simulink model "Thesis_VehicleModel_MPC_ECMS"  (R2018b)
settings: Solver=FixedStepAuto  StartTime=0.0  StopTime=10  FixedStep=0.01  RelTol=1e-5
PostLoadFcn:
  | , if any(exist('dsrtsu_mdlpostloadfcn', 'file') == [2, 3, 6]), try dsrtsu_mdlpostloadfcn('Execute', bdroot); catch fprintf('Error in PostLoadFcn (dsrtsu_mdlpostloadfcn) for model "%s":\n %s\n', bdroot, lasterr); end, end,
InitFcn:
  | clc;clear all;
model workspace (MAT data in the model file):
  MDL.BatteryModel.AccyLoad = 600
  MDL.BatteryModel.Voc = 340
  MDL.BatteryModel.Rint = 0.08
  MDL.BatteryModel.Ecap = 8.8
  MDL.BatteryModel.SOCi = 0.5
  MDL.BrakeSys.MaxBrakeForce = 10000
  MDL.BrakeSys.RegenFraction = 0.55
  MDL.Driveline.TFRatio = 3.5
  MDL.Driveline.MaxTrac = 8000
  MDL.Driveline.BrakeGain = 500
  MDL.Driveline.Spinloss = 3.6
  MDL.EngineModel.C0 = 6760
  MDL.EngineModel.C1 = 1.32
  MDL.EngineModel.C2 = 4.2e-06
  MDL.EngineModel.LHV = 44400
  MDL.EngineModel.MaxOutPwr = 73000
  MDL.EngineModel.EngStartEnergy = 0
  MDL.EngineModel.AccyLoad = 600
  MDL.EngineModel.EffMapData = [800  800  800  800  800  800  800  800  800  800; 700  700  700  700  700  700  700  700  700  700; 600  600  600  600  600  600  600  600  600  600; 400  400  400  400  400  400  400  400  400  400; 275  275  275  275  275  275  278  280  285  290; 255  255  255  255  255  258  260  265  270  275; 245  244  243  243  244  245  248  250  260  265; 235  234  234  236  238  239  240  242  246  252; 225  222  221  223  226  228  230  232  242  247; 225  223  220  215  218  221  225  232  240  244; 227  226  221  216  218  220  226  232  242  244; 230  228  226  225  222  224  226  232  240  243; 235  234  228  226  226  227  229  234  241  244; 240  237  234  230  228  229  230  235  240  244; 245  242  240  235  232  231  235  240  242  244; 248  246  244  242  234  235  241  246  250  252]
  MDL.EngineModel.EffMapRPM = [800 1000 1500 2000 2500 3000 3500 4000 4500 5000]
  MDL.EngineModel.EffMapTorque = [0 10 20 30 40 50 60 70 80 90 100 110 120 130 135 150]
  MDL.GeneratorModel.C0 = 600
  MDL.GeneratorModel.C1 = 0.033
  MDL.GeneratorModel.C2 = 8e-07
  MDL.GeneratorModel.PeakMechPwr = 50000
  MDL.GeneratorModel.ContMechPwr = 25000
  MDL.HVSCModel.TargetSOC = 0.45
  MDL.HVSCModel.SOC_gain = 100000
  MDL.LHV = 46400
  MDL.MotorModel.EtoWRatio = 0.98
  MDL.MotorModel.MaxPwrOut = 80000
  MDL.MotorModel.MaxTorque = 240
  MDL.MotorModel.MaxWhlSpd = 600
  MDL.MotorModel.EffMapTorque = [0 50 75 100 125 150 175 200 240]
  MDL.MotorModel.EffMapRPM = [0 500 1000 1250 1500 1750 2000 2250 2500 2750 3000 3250 3500 3750 4000 4250 4500 5000]
  MDL.MotorModel.EffMapData = [0.8  0.815  0.82  0.825  0.83  0.83  0.84  0.84  0.84  0.84  0.84  0.84  0.84  0.83  0.82  0.81  0.8  0.76; 0.83  0.87  0.9  0.865  0.88  0.92  0.92  0.92  0.92  0.92  0.92  0.92  0.92  0.915  0.9  0.86  0.85  0.82; 0.83  0.88  0.94  0.945  0.948  0.95  0.96  0.96  0.96  0.956  0.95  0.95  0.948  0.946  0.945  0.938  0.9  0.85; 0.82  0.88  0.94  0.948  0.95  0.96  0.96  0.96  0.96  0.96  0.96  0.96  0.95  0.955  0.95  0.945  0.94  0.86; 0.81  0.88  0.94  0.95  0.958  0.96  0.96  0.96  0.96  0.96  0.96  0.96  0.958  0.954  0.952  0.952  0.948  0.9; 0.81  0.86  0.94  0.95  0.95  0.95  0.95  0.95  0.95  0.95  0.95  0.95  0.95  0.96  0.95  0.948  0.94  0.94; 0.8  0.886  0.91  0.94  0.945  0.948  0.946  0.944  0.944  0.948  0.947  0.946  0.9455  0.945  0.944  0.943  0.942  0.941; 0.79  0.84  0.9  0.92  0.93  0.94  0.94  0.94  0.94  0.94  0.94  0.94  0.94  0.94  0.94  0.94  0.94  0.94; 0.77  0.81  0.86  0.86  0.86  0.86  0.86  0.86  0.86  0.86  0.86  0.86  0.86  0.86  0.86  0.86  0.86  0.86]
  MDL.Tire.Miu = 0.9
  MDL.Tire.Caf = 39000
  MDL.Tire.Car = 39000
  MDL.Tire.ContactPatch = 0.0003
  MDL.Tire.EffectiveRadius = 0.31
  MDL.Tire.Inertia = 0.9182
  MDL.Tire.c_rr = 0.01
  MDL.Tire.RelaxationLength = 0.248
  MDL.VehicleDynamics.M = 1500
  MDL.VehicleDynamics.Mi = 1560
  MDL.VehicleDynamics.CdA = 0.76
  MDL.VehicleDynamics.rho = 1.2
  MDL.VehicleDynamics.grade = 0
  MDL.VehicleDynamics.g = 9.81
  MDL.VehicleDynamics.V_i = 0
  MDL.VehicleDynamics.FrontLength = 1.524
  MDL.VehicleDynamics.RearLength = 1.2192
  MDL.VehicleDynamics.WheelBase = 2.7432
  MDL.VehicleDynamics.Inertia = 3000
  MDL.VehicleDynamics.HeightofCD = 0.32
  MDL.VehicleDynamics.HeightofCG = 0.3
  MDL.ThrottleController.KFA = [0  1; -0.3425  -5.0685]
  MDL.ThrottleController.KFB = [0; 904.1096]
  MDL.ThrottleController.KFC = [1 0]
  MDL.ThrottleController.KFL = [3.2; -0.2946]
values from neighbouring files (symbols this model uses):
  MDL =     [MDL.mat]
libraries: simulink x14, rtican x9, autolibshared x1, mpclib x1
(part 1 of 5)
settings Model: DSRTSU_INTERNAL_RTI_VER=510  DSRTSU_INTERNAL_RTI_TYPE=rti1006  RTICANMMDATA=struct('GeneralSetupData',struct('modelroot','C:\Users\UWECOCAR3\Desktop\YD_Thesis_dSPACE_Model','generalsettings',struct('filesettings',struct('destfolder',struct('Name','RTICANMM_FILES','Check',1),'buildfolder',struct('Name','.','Check',1),'AbsDestfolder',struct('Name','C:\Users\UWECOCAR3\Desktop\YD_Thesis_dSPACE_Model\RTICANMM_FILES'),'AbsBuildfolder',struct('Name','C:\Users\UWECOCAR3\Desktop\YD_Thesis_dSPACE_Model'))),'options',struct('addpaths',1,'rmpaths',1,'addtrcexclusion',logical(1),'cannavigator',struct('checkmonitoring',0),'show_usrtrc',0,'use_usrtrc',0),'advanced',struct('options',[1 1 1 1 1 1 1 1 1 1 1 1 1 1 1 1 1 1 1 1 1 1 1 1 1 1 1 1 1 1 1 1 1 1 1 1 1 1 1 1 1 1 1 1 1 1 1 1 1 1 1 1 1 1 1 1 1 1 1 1 1 1 1 1 1 1 1 1 1 1 1 1 1 1 1 1 1 1 1 1 1 1 1 1 1 1 1 1 1 1 1 1 1 1 1 1 1 1 1 1]),'MPSetup',{{}},'modelname','Thesis_VehicleModel_Integrate_Powertrain_17b','block','Thesis_VehicleModel_Integrate_Powertrain_17b'))  DSRTSU_INTERNAL_RTIFLEXRAYCONFIG=110  DSRTSU_INTERNAL_RTIFPGA=110  Creator=lyd21  LastModifiedBy=lyd21
settings SolverCC: ZeroCrossAlgorithm=Adaptive
settings OptimizationCC: BlockReduction=off
settings DebuggingCC: MaxConsecutiveZCsMsg=none  IgnoredZcDiagnostic=none
settings HardwareCC: ProdBitPerPointer=32  ProdBitPerSizeT=32  ProdBitPerPtrDiffT=32  ProdLargestAtomicInteger=Integer  ProdWordSize=32  ProdHWDeviceType=Custom Processor->Custom  TargetIntDivRoundTo=Zero  TargetEndianess=LittleEndian  TargetHWDeviceType=Custom Processor->Custom
settings SFSimCC: SimUseLocalCustomCode=off  MATLABDynamicMemAlloc=off
settings RTWCC: Description=Generic Real-Time Target  RTWUseLocalCustomCode=off
settings GRTTargetCC: TargetLangStandard=C89/C90 (ANSI)

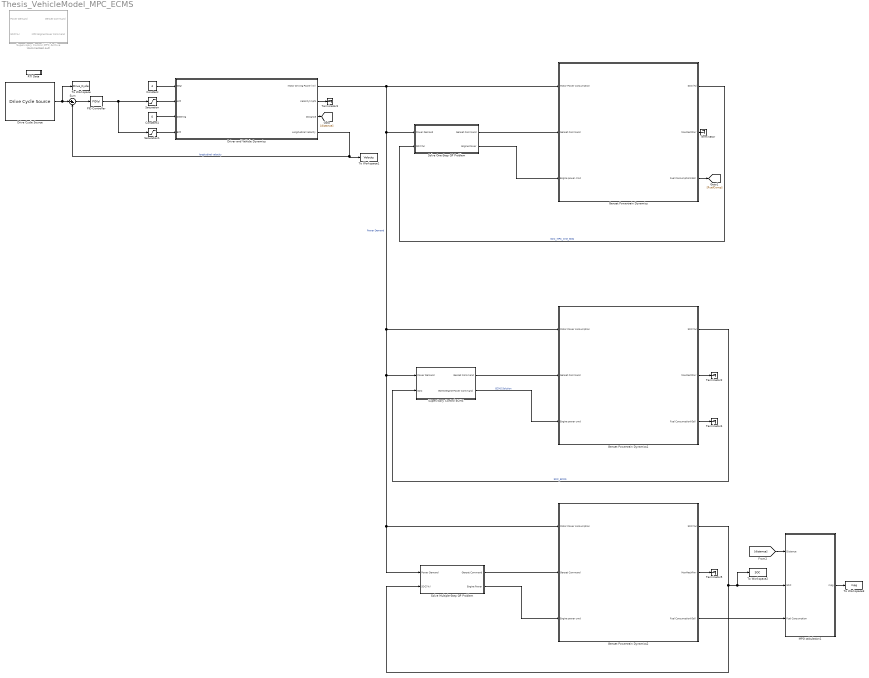
== system Thesis_VehicleModel_MPC_ECMS ==
  Constant : Constant  Value=4
  Constant1 : Constant  Value=0
  Drive Cycle Source : autolibshared/Drive Cycle Source  cycleVar=FTP72  fileVar=C:\Users\lyd21\OneDrive\Documents\MATLAB\Thesis_Model_Winter\TEST_CTY_HWY.mat  tfinal="1372  seconds"  cycleRepeat=off  outAccPort=off  outGearPort=off  gearList=No gear data  t_wot1=5  xdot_woto=0  xdot_wot1=30  t_wot2=20  xdot_wot2=0  t_wotend=30  srcUnit=m/s  outUnit=m/s  srcAccUnit=m/s/s  outAccUnit=m/s^2  dt=0  aMode=1
      settings: SourceProductName=Powertrain Blockset  SourceProductBaseCode=PW
  "Driver and Vehicle Dynamics " : Subsystem
  Genset Powertrain Dynamics : Subsystem
  Genset Powertrain Dynamics1 : Subsystem
  Genset Powertrain Dynamics2 : Subsystem
  MPG calculation1 : Subsystem
  PID Controller : simulink/Continuous/PID Controller  Controller=PID  Form=Parallel  TimeDomain=Continuous-time  SampleTime=-1  IntegratorMethod=Forward Euler  FilterMethod=Forward Euler  ControllerParametersSource=internal  P=1  I=0  D=0  UseFilter=on  N=100  TunerSelectOption=Transfer Function Based (PID Tuner App)  InitialConditionSource=internal  InitialConditionForIntegrator=0  InitialConditionForFilter=0  DifferentiatorICPrevScaledInput=0  ExternalReset=none  TrackingMode=off  Kt=1  LimitOutput=off  UpperSaturationLimit=inf  LowerSaturationLimit=-inf  LinearizeAsGain=on  AntiWindupMode=none  Kb=1  POutMin=[]  POutMax=[]  IOutMin=[]  IOutMax=[]  DOutMin=[]  DOutMax=[]  NOutMin=[]  NOutMax=[]  SumOutMin=[]  SumOutMax=[]  SaturationOutMin=[]  SaturationOutMax=[]  PParamMin=[]  PParamMax=[]  IParamMin=[]  IParamMax=[]  DParamMin=[]  DParamMax=[]  NParamMin=[]  NParamMax=[]  KbParamMin=[]  KbParamMax=[]  KtParamMin=[]  KtParamMax=[]  KbOutMin=[]  KbOutMax=[]  KtOutMin=[]  KtOutMax=[]  IntegratorOutMin=[]  IntegratorOutMax=[]  FilterOutMin=[]  FilterOutMax=[]  SumI1OutMin=[]  SumI1OutMax=[]  SumI2OutMin=[]  SumI2OutMax=[]  SumI3OutMin=[]  SumI3OutMax=[]  SumI4OutMin=[]  SumI4OutMax=[]  SumDOutMin=[]  SumDOutMax=[]  DifferentiatorOutMin=[]  DifferentiatorOutMax=[]  FilterDiffOutCoefMin=[]  FilterDiffOutCoefMax=[]  ReciprocalOutMin=[]  ReciprocalOutMax=[]  SumDenOutMin=[]  SumDenOutMax=[]  SumNumOutMin=[]  SumNumOutMax=[]  DivideOutMin=[]  DivideOutMax=[]  IntegratorContinuousStateAttributes=''  IntegratorStateMustResolveToSignalObject=off  IntegratorRTWStateStorageClass=Auto  FilterContinuousStateAttributes=''  FilterStateMustResolveToSignalObject=off  FilterRTWStateStorageClass=Auto  ParallelPVariant=InternalParameters  IdealPVariant=Disabled  IVariant=InternalParameters  DVariant=InternalParameters  IntegratorVariant=Continuous  SatVariant=Disabled  AWVariant=Passthrough  PCopyVariant=Disabled  TRVariant=Disabled  FdbkBlocksVariant=Forward  IdealPFdbkVariant=Disabled  SatFdbkVariant=Disabled  DerivativeFilterVariant=ContFilter  NVariant=InternalParameters  NCopyVariant=Disabled  FilterICVariant=InternalICsFilter  IntegratorICVariant=InternalICs  ExternalResetVariant=Disabled  TRSumVariant=Passthrough  SumFdbkVariant=Disabled  SumVariant=Sum_PID
  RTI Data : Subsystem  Tag=struct('RTIDataServer',struct('RTIDataServerVs','2','RTIModelDescription','struct(''main'',''Thesis_VehicleModel_Integrate_Powertrain_ETAS_17b'',''sub'','''',''isMp'',0)'))  LoadFcn="if exist('rtidc'), try,  rtidc('DataHostBlockClbLoad', gcbh); catch, disp(['Warning: ''LoadFcn'' for RTI Data block failed: ' lasterr]); end, end,"  mask(RTI_DATA_HOST){}
      mask help:
      | RTI Data Block.
      | This block is used by RTI to store internal model-dependent data.
      | Please keep this block on the root level of the model. Deleting this block will result in data loss.
      |
      | NEVER DELETE OR COPY THIS BLOCK!
      settings: CopyFcn="if exist('rtidc'), try,  rtidc('DataHostBlockClbCopy', gcbh); catch, disp(['Warning: ''CopyFcn'' for RTI Data block failed: ' lasterr]); end, end,"  DeleteFcn="if exist('rtidc'), try,  rtidc('DataHostBlockClbDelete', gcbh); catch, disp(['Warning: ''DeleteFcn'' for RTI Data block failed: ' lasterr]); end, end,"  ModelCloseFcn="if exist('rtidc'), try,  rtidc('DataHostBlockClbModelClose', gcbh); catch, disp(['Warning: ''ModelCloseFcn'' for RTI Data block failed: ' lasterr]); end, end,"  PreSaveFcn="if exist('rtidc'), try,  rtidc('DataHostBlockClbPreSave', gcbh); catch, disp(['Warning: ''PreSaveFcn'' for RTI Data block failed: ' lasterr]); end, end,"  PostSaveFcn="if exist('rtidc'), try,  rtidc('DataHostBlockClbPostSave', gcbh); catch, disp(['Warning: ''PostSaveFcn'' for RTI Data block failed: ' lasterr]); end, end,"  NameChangeFcn="if exist('rtidc'), try,  rtidc('DataHostBlockClbNameChange', gcbh); catch, disp(['Warning: ''NameChangeFcn'' for RTI Data block failed: ' lasterr]); end, end,"
      mask Help:
      | RTI Data Block.
      | This block is used by RTI to store internal model-dependent data.
      | Please keep this block on the root level of the model. Deleting this block will result in data loss.
      | 
      | NEVER DELETE OR COPY THIS BLOCK!
      mask Display:
      | text(0.5, 0.5, 'RTI Data', 'HorizontalAlignment', 'center');
      | plot([1 0]);
  Saturation : Saturate  UpperLimit=0.98  LowerLimit=0
  Saturation1 : Saturate  UpperLimit=0  LowerLimit=-1
  Solve Multiple-Step QP Problem : Subsystem
  Solve One-Step QP Problem : Subsystem
  Sum : Sum  Inputs=|+-
  Supervisory Control ECMS : Subsystem
  Supervisory Control MPC Archive : Subsystem  Commented=on
  Terminator{,2..5} (5 alike) : Terminator
  To Workspace : ToWorkspace  VariableName=Drive_Cycle  SampleTime=-1
  To Workspace1 : ToWorkspace  VariableName=Velocity  SampleTime=-1
  To Workspace2 : ToWorkspace  VariableName=SOC  SampleTime=-1
  To Workspace3 : ToWorkspace  VariableName=mpg  SampleTime=-1
  wires:
  Genset Powertrain Dynamics/1(SOC(%)) -> Solve One-Step QP Problem/2(SOC(%))  "SOC_MPC_One_Step"
  "Driver and Vehicle Dynamics "/1("Motor Driving Power (W) ") -> Genset Powertrain Dynamics/1(Motor Power consumption), Solve One-Step QP Problem/1(Power Demand), Genset Powertrain Dynamics2/1(Motor Power consumption), Solve Multiple-Step QP Problem/1(Power Demand), Supervisory Control ECMS/1(Power Demand), Genset Powertrain Dynamics1/1(Motor Power consumption)  "Power Demand"
  Genset Powertrain Dynamics/3(Fuel Consumption(Gal)) -> [FuelComp]
  Saturation/1 -> "Driver and Vehicle Dynamics "/2(APP)
  Constant/1 -> "Driver and Vehicle Dynamics "/1(Gear)
  Constant1/1 -> "Driver and Vehicle Dynamics "/3(Steering)
  Solve One-Step QP Problem/1(Genset Command) -> Genset Powertrain Dynamics/2(Genset Command)
  Sum/1 -> PID Controller/1
  Drive Cycle Source/1 -> To Workspace/1, Sum/1
  "Driver and Vehicle Dynamics "/4(Longitudinal Velocity) -> Sum/2, To Workspace1/1  "longitudinal velocity"
  PID Controller/1 -> Saturation1/1, Saturation/1
  "Driver and Vehicle Dynamics "/3(Distance) -> [distance]
  Saturation1/1 -> "Driver and Vehicle Dynamics "/4(BPP)
  "Driver and Vehicle Dynamics "/2(Velocity(mph)) -> Terminator3/1
  Solve One-Step QP Problem/2("Engine Power ") -> Genset Powertrain Dynamics/3(Engine power cmd)
  Genset Powertrain Dynamics/2(MaxMechPwr) -> Terminator/1
  Genset Powertrain Dynamics1/1(SOC(%)) -> Supervisory Control ECMS/2(SOC)  "SOC_ECMS"
  Genset Powertrain Dynamics1/2(MaxMechPwr) -> Terminator2/1
  Genset Powertrain Dynamics1/3(Fuel Consumption(Gal)) -> Terminator4/1
  Supervisory Control ECMS/1(Genset Command) -> Genset Powertrain Dynamics1/2(Genset Command)
  Supervisory Control ECMS/2(ECMS Engine Power Command) -> Genset Powertrain Dynamics1/3(Engine power cmd)  "ECMS Solution"
  Solve Multiple-Step QP Problem/1(Genset Command) -> Genset Powertrain Dynamics2/2(Genset Command)
  Solve Multiple-Step QP Problem/2("Engine Power ") -> Genset Powertrain Dynamics2/3(Engine power cmd)
  Genset Powertrain Dynamics2/2(MaxMechPwr) -> Terminator5/1
  Genset Powertrain Dynamics2/1(SOC(%)) -> Solve Multiple-Step QP Problem/2(SOC(%)), To Workspace2/1, MPG calculation1/2("SOC ")
  MPG calculation1/1(mpg) -> To Workspace3/1
  [distance] -> MPG calculation1/1(Distance)
  Genset Powertrain Dynamics2/3(Fuel Consumption(Gal)) -> MPG calculation1/3(Fuel Consumption)

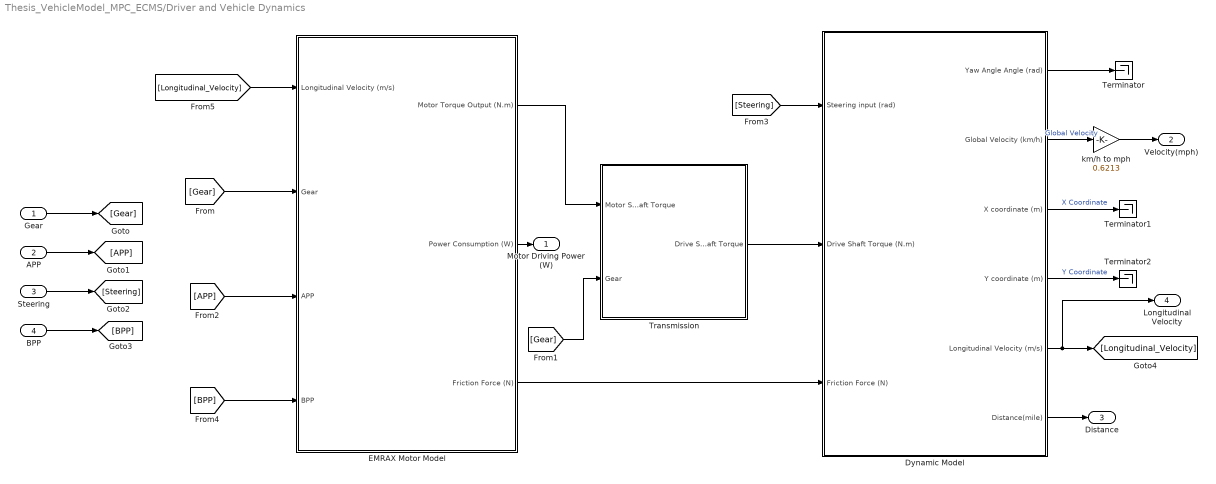
== system Thesis_VehicleModel_MPC_ECMS/Driver and Vehicle Dynamics  ==
  Gear : Inport
  APP : Inport  Port=2
  Steering : Inport  Port=3
  BPP : Inport  Port=4
  Dynamic Model : Subsystem
  "EMRAX Motor Model " : Subsystem
  Terminator : Terminator
  Terminator1 : Terminator
  Terminator2 : Terminator
  Transmission : Subsystem
  km/h to mph : Gain  Gain=0.6213
  "Motor Driving Power (W) " : Outport
  Velocity(mph) : Outport  Port=2
  Distance : Outport  Port=3
  Longitudinal Velocity : Outport  Port=4
  wires:
  Dynamic Model/1(Yaw Angle Angle (rad)) -> Terminator/1
  Dynamic Model/4(Y coordinate (m)) -> Terminator2/1  "Y Coordinate"
  "EMRAX Motor Model "/1(Motor Torque Output (N.m)) -> Transmission/1("Motor Shaft Torque ")
  [Gear] -> Transmission/2(Gear)
  Transmission/1(Drive Shaft Torque) -> Dynamic Model/2(Drive Shaft Torque (N.m))
  [Gear] -> "EMRAX Motor Model "/2("Gear ")
  [APP] -> "EMRAX Motor Model "/3(APP)
  [Steering] -> Dynamic Model/1(Steering input (rad))
  Dynamic Model/2(Global Velocity (km/h)) -> km/h to mph/1  "Global Velocity"
  [BPP] -> "EMRAX Motor Model "/4(BPP)
  "EMRAX Motor Model "/3("Friction Force (N) ") -> Dynamic Model/3(Friction Force (N))
  "EMRAX Motor Model "/2(Power Consumption (W)) -> "Motor Driving Power (W) "/1
  [Longitudinal_Velocity] -> "EMRAX Motor Model "/1(Longitudinal Velocity (m/s))
  Dynamic Model/3(X coordinate (m)) -> Terminator1/1  "X Coordinate"
  Gear/1 -> [Gear]
  APP/1 -> [APP]
  Steering/1 -> [Steering]
  BPP/1 -> [BPP]
  Dynamic Model/6(Distance(mile)) -> Distance/1
  km/h to mph/1 -> Velocity(mph)/1
  Dynamic Model/5(Longitudinal Velocity (m/s)) -> Longitudinal Velocity/1, [Longitudinal_Velocity]

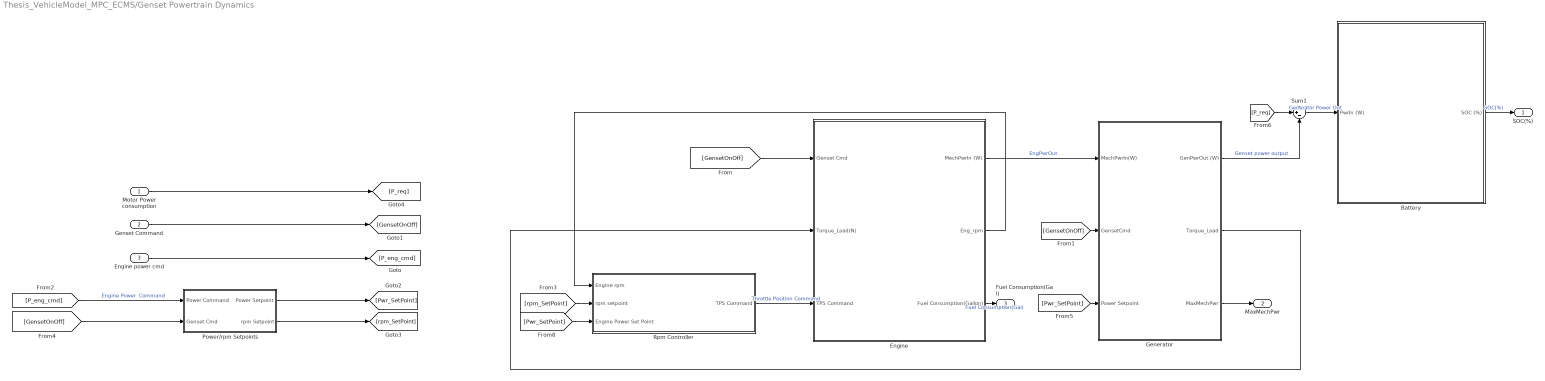
== system Thesis_VehicleModel_MPC_ECMS/Genset Powertrain Dynamics ==
  Motor Power consumption : Inport
  Genset Command : Inport  Port=2
  Engine power cmd : Inport  Port=3
  Battery : Subsystem
  Engine : Subsystem
  Generator : Subsystem
  Power/rpm Setpoints : Subsystem
  Rpm Controller : Subsystem
  Sum1 : Sum  Inputs=|+-
  SOC(%) : Outport
  MaxMechPwr : Outport  Port=2
  Fuel Consumption(Gal) : Outport  Port=3
  wires:
  Generator/2("Torque_Load ") -> Engine/2("Torque_Load(N) ")
  [P_req] -> Sum1/1
  Engine/1(MechPwrIn (W)) -> Generator/1(MechPwrIn(W))  "EngPwrOut"
  Sum1/1 -> Battery/1(PwrIn (W))  "Generator Power Out"
  Battery/1(SOC (%)) -> SOC(%)/1  "SOC(%)"
  Generator/1(GenPwrOut (W)) -> Sum1/2  "Genset power output"
  Generator/3(MaxMechPwr) -> MaxMechPwr/1
  Rpm Controller/1(TPS Command) -> Engine/3(TPS Command)  "Throttle Position Command"
  Engine/2("Eng_rpm ") -> Rpm Controller/1(Engine rpm)
  Engine power cmd/1 -> [P_eng_cmd]
  Genset Command/1 -> [GensetOnOff]
  [GensetOnOff] -> Engine/1(Genset Cmd)
  [GensetOnOff] -> Generator/2(GensetCmd)
  Power/rpm Setpoints/1(Power Setpoint) -> [Pwr_SetPoint]
  Power/rpm Setpoints/2(rpm Setpoint) -> [rpm_SetPoint]
  [rpm_SetPoint] -> Rpm Controller/2(rpm setpoint)
  [Pwr_SetPoint] -> Generator/3(Power Setpoint)
  Motor Power consumption/1 -> [P_req]
  Engine/3(Fuel Consumption(Gallon)) -> Fuel Consumption(Gal)/1  "Fuel Consumption(Gal)"
  [P_eng_cmd] -> Power/rpm Setpoints/1(Power Command)  "Engine Power  Command"
  [Pwr_SetPoint] -> Rpm Controller/3(Engine Power Set Point)
  [GensetOnOff] -> Power/rpm Setpoints/2(Genset Cmd)

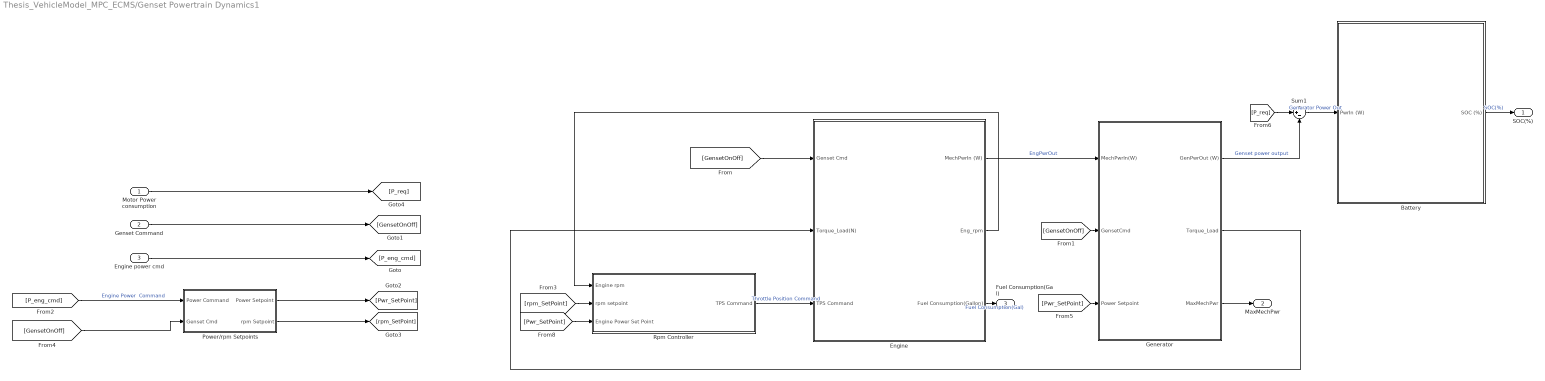
== system Thesis_VehicleModel_MPC_ECMS/Genset Powertrain Dynamics1 ==
  Motor Power consumption : Inport
  Genset Command : Inport  Port=2
  Engine power cmd : Inport  Port=3
  Battery : Subsystem
  Engine : Subsystem
  Generator : Subsystem
  Power/rpm Setpoints : Subsystem
  Rpm Controller : Subsystem
  Sum1 : Sum  Inputs=|+-
  SOC(%) : Outport
  MaxMechPwr : Outport  Port=2
  Fuel Consumption(Gal) : Outport  Port=3
  wires:
  Generator/2("Torque_Load ") -> Engine/2("Torque_Load(N) ")
  [P_req] -> Sum1/1
  Engine/1(MechPwrIn (W)) -> Generator/1(MechPwrIn(W))  "EngPwrOut"
  Sum1/1 -> Battery/1(PwrIn (W))  "Generator Power Out"
  Battery/1(SOC (%)) -> SOC(%)/1  "SOC(%)"
  Generator/1(GenPwrOut (W)) -> Sum1/2  "Genset power output"
  Generator/3(MaxMechPwr) -> MaxMechPwr/1
  Rpm Controller/1(TPS Command) -> Engine/3(TPS Command)  "Throttle Position Command"
  Engine/2("Eng_rpm ") -> Rpm Controller/1(Engine rpm)
  Engine power cmd/1 -> [P_eng_cmd]
  Genset Command/1 -> [GensetOnOff]
  [GensetOnOff] -> Engine/1(Genset Cmd)
  [GensetOnOff] -> Generator/2(GensetCmd)
  Power/rpm Setpoints/1(Power Setpoint) -> [Pwr_SetPoint]
  Power/rpm Setpoints/2(rpm Setpoint) -> [rpm_SetPoint]
  [rpm_SetPoint] -> Rpm Controller/2(rpm setpoint)
  [Pwr_SetPoint] -> Generator/3(Power Setpoint)
  Motor Power consumption/1 -> [P_req]
  Engine/3(Fuel Consumption(Gallon)) -> Fuel Consumption(Gal)/1  "Fuel Consumption(Gal)"
  [P_eng_cmd] -> Power/rpm Setpoints/1(Power Command)  "Engine Power  Command"
  [Pwr_SetPoint] -> Rpm Controller/3(Engine Power Set Point)
  [GensetOnOff] -> Power/rpm Setpoints/2(Genset Cmd)

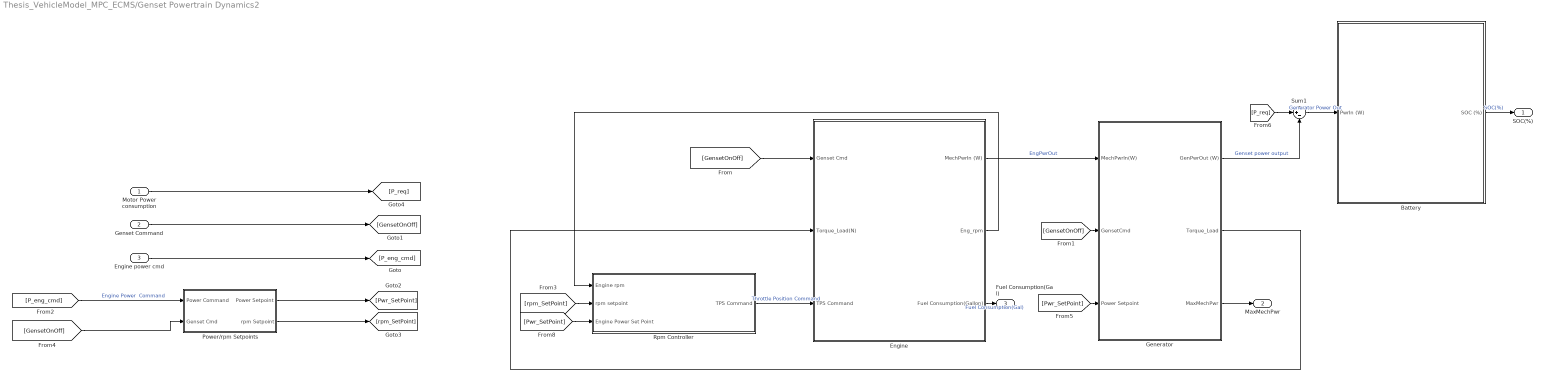
== system Thesis_VehicleModel_MPC_ECMS/Genset Powertrain Dynamics2 ==
  Motor Power consumption : Inport
  Genset Command : Inport  Port=2
  Engine power cmd : Inport  Port=3
  Battery : Subsystem
  Engine : Subsystem
  Generator : Subsystem
  Power/rpm Setpoints : Subsystem
  Rpm Controller : Subsystem
  Sum1 : Sum  Inputs=|+-
  SOC(%) : Outport
  MaxMechPwr : Outport  Port=2
  Fuel Consumption(Gal) : Outport  Port=3
  wires:
  Generator/2("Torque_Load ") -> Engine/2("Torque_Load(N) ")
  [P_req] -> Sum1/1
  Engine/1(MechPwrIn (W)) -> Generator/1(MechPwrIn(W))  "EngPwrOut"
  Sum1/1 -> Battery/1(PwrIn (W))  "Generator Power Out"
  Battery/1(SOC (%)) -> SOC(%)/1  "SOC(%)"
  Generator/1(GenPwrOut (W)) -> Sum1/2  "Genset power output"
  Generator/3(MaxMechPwr) -> MaxMechPwr/1
  Rpm Controller/1(TPS Command) -> Engine/3(TPS Command)  "Throttle Position Command"
  Engine/2("Eng_rpm ") -> Rpm Controller/1(Engine rpm)
  Engine power cmd/1 -> [P_eng_cmd]
  Genset Command/1 -> [GensetOnOff]
  [GensetOnOff] -> Engine/1(Genset Cmd)
  [GensetOnOff] -> Generator/2(GensetCmd)
  Power/rpm Setpoints/1(Power Setpoint) -> [Pwr_SetPoint]
  Power/rpm Setpoints/2(rpm Setpoint) -> [rpm_SetPoint]
  [rpm_SetPoint] -> Rpm Controller/2(rpm setpoint)
  [Pwr_SetPoint] -> Generator/3(Power Setpoint)
  Motor Power consumption/1 -> [P_req]
  Engine/3(Fuel Consumption(Gallon)) -> Fuel Consumption(Gal)/1  "Fuel Consumption(Gal)"
  [P_eng_cmd] -> Power/rpm Setpoints/1(Power Command)  "Engine Power  Command"
  [Pwr_SetPoint] -> Rpm Controller/3(Engine Power Set Point)
  [GensetOnOff] -> Power/rpm Setpoints/2(Genset Cmd)

== system Thesis_VehicleModel_MPC_ECMS/MPG calculation1 ==
  Distance : Inport
  "SOC " : Inport  Port=2
  Fuel Consumption : Inport  Port=3
  Average Efficiency : Gain  Gain=1/0.25
  Constant : Constant  Value=MDL.BatteryModel.SOCi
  Divide : Product  Inputs=*/
  Gain : Gain  Gain=0.01
  Gain3 : Gain  Gain=MDL.BatteryModel.Ecap*3600*1000
  Gain4 : Gain  Gain=1/MDL.EngineModel.LHV
  Rate Transition : RateTransition
  Saturation : Saturate  UpperLimit=inf  LowerLimit=0.01
  Subtract : Sum  Inputs=+-
  Sum : Sum  Inputs=|++
  g to gal : Gain  Gain=0.77/1000/3.785
  mpg : Outport
  wires:
  Divide/1 -> Rate Transition/1
  Fuel Consumption/1 -> Sum/1
  Distance/1 -> Divide/1
  "SOC "/1 -> Gain/1
  Constant/1 -> Subtract/2
  Subtract/1 -> Gain3/1
  Saturation/1 -> Divide/2  "Equivalent Fuel Consumption (gal)"
  g to gal/1 -> Average Efficiency/1
  Gain4/1 -> g to gal/1
  Gain3/1 -> Gain4/1
  Gain/1 -> Subtract/1
  Average Efficiency/1 -> Sum/2  "0.5859*(SOC - SOC_ref)"
  Sum/1 -> Saturation/1
  Rate Transition/1 -> mpg/1  "mpg"

== system Thesis_VehicleModel_MPC_ECMS/RTI Data ==
  RTI Data Store : Subsystem  Tag="struct('private',struct('version',struct('dsVer',uint32(2),'dsVerCreation',uint32(2),'RTI',struct('ver','7.9','type','RTI1006')),'access',struct('type','Model','isPerm',1,'created',['07-Dec-2018 11:10:24'],'modified',['10-Dec-2018 15:20:08'],'location','')),'public',struct('main',struct('data',[]),'sub',struct('name',{{'Thesis_VehicleModel_Integrate_Powertrain_ETAS_17b'}},'data',{{struct('TH',struct('thTaskInfo',struct('taskType',{'TIMER','HWINT','TMRINT','SWINT','GLINT'},'tasksNumOf',{1,0,0,0,0},'srcIds',{{'TIMERA'},{},{},{},{}},'taskNames',{{['Timer Task 1']},{},{},{},{}})),'th_tc',struct('dataType','TASK','taskGroupId','','taskGroupList',{{}},'taskSchedulingPolicy','FCFS','taskType','TIMER','blkh',-1,'srcId','TIMERA','srcSgnName',['Timer A interrupt'],'srcCpuName','','taskName',['Timer Task 1  [0.01] s'],'taskNameDisplayExt','','smplTime',0.01,'smplTimeOffs',0,'hasFixedPriority',0,'priority',1,'hasFixedOvc',0,'ovcType',1,'ovcMax',1),'tc_th',struct('dataType','TASK','taskGroupId','','taskGroupList',{{}},'taskSchedulingPolicy','FCFS','taskType','TIMER','blkh',-1,'srcId','TIMERA','srcSgnName',['Timer A interrupt'],'srcCpuName','','taskName',['Timer Task 1  [0.01] s'],'taskNameDisplayExt','','smplTime',0.01,'smplTimeOffs',0,'hasFixedPriority',0,'priority',1,'hasFixedOvc',0,'ovcType',1,'ovcMax',1))}})))"  mask(RTI_DATA_STORE){}
      mask help:
      | RTI Data Store Block. This block is used by RTI to store internal model dependent data. Deleting this block will result in data loss.
      |
      | NEVER DELETE, COPY, OR MODIFY THIS BLOCK!
      mask Help:
      | RTI Data Store Block. This block is used by RTI to store internal model dependent data. Deleting this block will result in data loss.
      | 
      | NEVER DELETE, COPY, OR MODIFY THIS BLOCK!
      mask Display: text(0.5, 0.5, ' ', 'HorizontalAlignment', 'center');

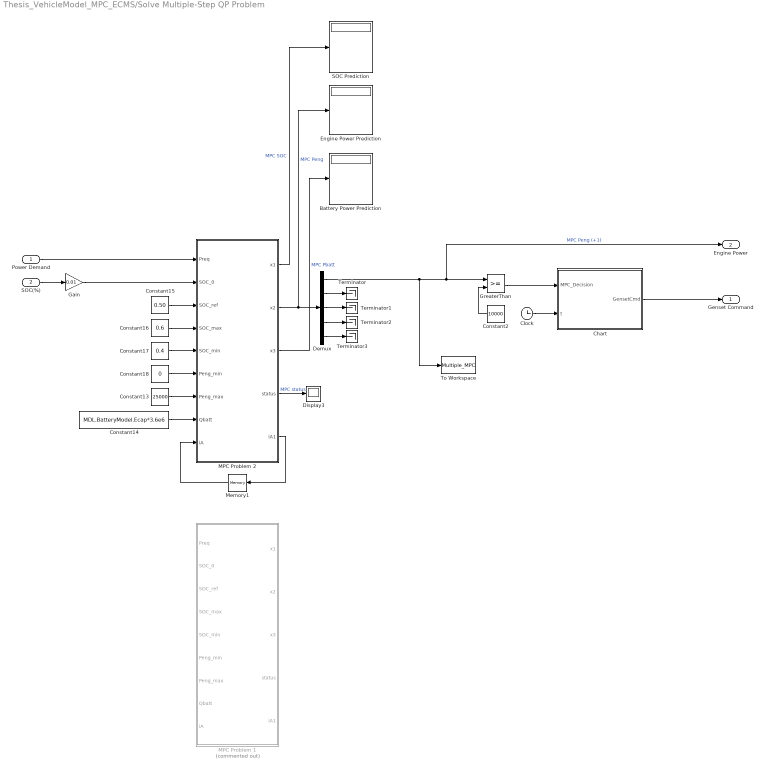
== system Thesis_VehicleModel_MPC_ECMS/Solve Multiple-Step QP Problem ==
  Power Demand : Inport
  SOC(%) : Inport  Port=2
  Battery Power Prediction : Display
  Chart : Stateflow chart  TreatAsAtomicUnit=on
  Clock : Clock
  Constant13 : Constant  Value=25000
  Constant14 : Constant  Value=MDL.BatteryModel.Ecap*3.6e6
  Constant15 : Constant  Value=0.50
  Constant16 : Constant  Value=0.6
  Constant17 : Constant  Value=0.4
  Constant18 : Constant  Value=0
  Constant2 : Constant  Value=10000
  Demux : Demux  Outputs=5
  Display3 : Display
  Engine Power Prediction : Display
  Gain : Gain  Gain=0.01
  GreaterThan : RelationalOperator  OutDataTypeStr=boolean  RndMeth=Simplest
  MPC Problem 1 : MATLAB Function  Commented=on  TreatAsAtomicUnit=on
  MPC Problem 2 : MATLAB Function  TreatAsAtomicUnit=on
  Memory1 : Memory  InitialCondition=false(30,1)
  SOC Prediction : Display
  Terminator{,1..3} (4 alike) : Terminator
  To Workspace : ToWorkspace  VariableName=Multiple_MPC  SampleTime=-1
  Genset Command : Outport
  "Engine Power " : Outport  Port=2
  wires:
  Chart/1(GensetCmd) -> Genset Command/1
  Constant2/1 -> GreaterThan/2
  GreaterThan/1 -> Chart/1(MPC_Decision)
  Clock/1 -> Chart/2(t)
  SOC(%)/1 -> Gain/1
  Demux/1 -> To Workspace/1, GreaterThan/1, "Engine Power "/1  "MPC Peng (+1)"
  Constant15/1 -> MPC Problem 2/3(SOC_ref)
  Constant16/1 -> MPC Problem 2/4(SOC_max)
  Constant17/1 -> MPC Problem 2/5(SOC_min)
  Constant18/1 -> MPC Problem 2/6(Peng_min)
  Constant13/1 -> MPC Problem 2/7(Peng_max)
  Constant14/1 -> MPC Problem 2/8(Qbatt)
  MPC Problem 2/1(x1) -> SOC Prediction/1  "MPC SOC"
  MPC Problem 2/3(x3) -> Battery Power Prediction/1  "MPC Pbatt"
  MPC Problem 2/4(status) -> Display3/1  "MPC status"
  Memory1/1 -> MPC Problem 2/9(iA)
  MPC Problem 2/5(iA1) -> Memory1/1
  Gain/1 -> MPC Problem 2/2(SOC_0)
  Power Demand/1 -> MPC Problem 2/1(Preq)
  MPC Problem 2/2(x2) -> Demux/1, Engine Power Prediction/1  "MPC Peng"
  Demux/2 -> Terminator/1
  Demux/5 -> Terminator3/1
  Demux/4 -> Terminator2/1
  Demux/3 -> Terminator1/1

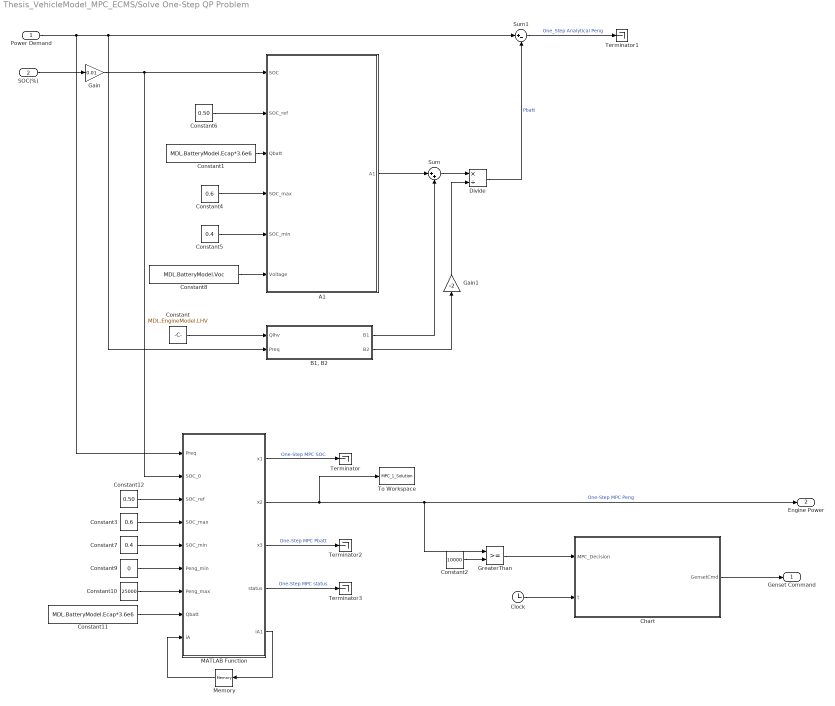
== system Thesis_VehicleModel_MPC_ECMS/Solve One-Step QP Problem ==
  Power Demand : Inport
  SOC(%) : Inport  Port=2
  A1 : MATLAB Function  TreatAsAtomicUnit=on
  "B1, B2" : MATLAB Function  TreatAsAtomicUnit=on
  Chart : Stateflow chart  TreatAsAtomicUnit=on
  Clock : Clock
  Constant : Constant  Value=MDL.EngineModel.LHV
  Constant1 : Constant  Value=MDL.BatteryModel.Ecap*3.6e6
  Constant10 : Constant  Value=25000
  Constant11 : Constant  Value=MDL.BatteryModel.Ecap*3.6e6
  Constant12 : Constant  Value=0.50
  Constant2 : Constant  Value=10000
  Constant3 : Constant  Value=0.6
  Constant4 : Constant  Value=0.6
  Constant5 : Constant  Value=0.4
  Constant6 : Constant  Value=0.50
  Constant7 : Constant  Value=0.4
  Constant8 : Constant  Value=MDL.BatteryModel.Voc
  Constant9 : Constant  Value=0
  Divide : Product  Inputs=*/
  Gain : Gain  Gain=0.01
  Gain1 : Gain  Gain=-2
  GreaterThan : RelationalOperator  OutDataTypeStr=boolean  RndMeth=Simplest
  MATLAB Function : MATLAB Function  TreatAsAtomicUnit=on
  Memory : Memory  InitialCondition=false(4,1)
  Sum : Sum  Inputs=|++
  Sum1 : Sum  Inputs=|+-
  Terminator{,1..3} (4 alike) : Terminator
  To Workspace : ToWorkspace  VariableName=MPC_1_Solution  SampleTime=-1
  Genset Command : Outport
  "Engine Power " : Outport  Port=2
  wires:
  "B1, B2"/1(B1) -> Sum/2
  A1/1(A1) -> Sum/1
  Sum/1 -> Divide/1
  "B1, B2"/2(B2) -> Gain1/1
  Divide/1 -> Sum1/2  "Pbatt"
  Constant/1 -> "B1, B2"/1(Qlhv)
  Constant5/1 -> A1/5(SOC_min)
  Constant6/1 -> A1/2(SOC_ref)
  Constant8/1 -> A1/6(Voltage)
  Constant4/1 -> A1/4(SOC_max)
  Constant1/1 -> A1/3(Qbatt)
  Chart/1(GensetCmd) -> Genset Command/1
  Constant2/1 -> GreaterThan/2
  GreaterThan/1 -> Chart/1(MPC_Decision)
  Clock/1 -> Chart/2(t)
  Gain1/1 -> Divide/2
  Power Demand/1 -> Sum1/1, "B1, B2"/2(Preq), MATLAB Function/1(Preq)
  SOC(%)/1 -> Gain/1
  Constant7/1 -> MATLAB Function/5(SOC_min)
  Constant3/1 -> MATLAB Function/4(SOC_max)
  Constant9/1 -> MATLAB Function/6(Peng_min)
  Constant10/1 -> MATLAB Function/7(Peng_max)
  Constant11/1 -> MATLAB Function/8(Qbatt)
  Constant12/1 -> MATLAB Function/3(SOC_ref)
  Sum1/1 -> Terminator1/1  "One_Step Analytical Peng"
  Gain/1 -> A1/1(SOC), MATLAB Function/2(SOC_0)
  MATLAB Function/5(iA1) -> Memory/1
  Memory/1 -> MATLAB Function/9(iA)
  MATLAB Function/4(status) -> Terminator3/1  "One-Step MPC status"
  MATLAB Function/1(x1) -> Terminator/1  "One-Step MPC SOC"
  MATLAB Function/2(x2) -> To Workspace/1, GreaterThan/1, "Engine Power "/1  "One-Step MPC Peng"
  MATLAB Function/3(x3) -> Terminator2/1  "One-Step MPC Pbatt"

== system Thesis_VehicleModel_MPC_ECMS/Supervisory Control ECMS ==
  Power Demand : Inport
  SOC : Inport  Port=2
  % to 1 : Gain  Gain=1/100
  Chart : Stateflow chart  TreatAsAtomicUnit=on
  Clock : Clock
  Constant : Constant  Value=MDL.EngineModel.LHV
  Constant1 : Constant  Value=MDL.BatteryModel.Ecap*3.6e6
  Constant4 : Constant  Value=0.6
  Constant5 : Constant  Value=0.4
  Constant6 : Constant  Value=0.50
  Constant7 : Constant
  Constant8 : Constant  Value=MDL.BatteryModel.Rint
  Constant9 : Constant  Value=10000
  GreaterThan : RelationalOperator  OutDataTypeStr=boolean  RndMeth=Simplest
  MATLAB Function : MATLAB Function  TreatAsAtomicUnit=on
  Terminator : Terminator
  To Workspace : ToWorkspace  VariableName=ECMS_Solution  SampleTime=-1
  Genset Command : Outport
  ECMS Engine Power Command : Outport  Port=2
  wires:
  Constant8/1 -> MATLAB Function/9(R)
  Constant1/1 -> MATLAB Function/4(Qbatt)
  MATLAB Function/1(Peng) -> To Workspace/1, ECMS Engine Power Command/1, GreaterThan/1  "ECMS Peng"
  Constant7/1 -> MATLAB Function/8(a)
  Constant6/1 -> MATLAB Function/7(SOCref)
  Constant5/1 -> MATLAB Function/6(SOCmin)
  Constant4/1 -> MATLAB Function/5(SOCmax)
  Constant/1 -> MATLAB Function/3(Qlhv)
  % to 1/1 -> MATLAB Function/2(SOCt)
  SOC/1 -> % to 1/1
  Chart/1(GensetCmd) -> Genset Command/1
  Constant9/1 -> GreaterThan/2
  GreaterThan/1 -> Chart/1(MPC_Decision)
  Clock/1 -> Chart/2(t)
  Power Demand/1 -> MATLAB Function/1(Preq)
  MATLAB Function/2(MinCost) -> Terminator/1  "ECMS Optimal Cost"

== system Thesis_VehicleModel_MPC_ECMS/Supervisory Control MPC Archive ==
  Power Demand : Inport
  "SOC(%) " : Inport  Port=2
  % to num : Gain  Gain=0.01
  Chart : Stateflow chart  TreatAsAtomicUnit=on
  Clock : Clock
  Constant : Constant  Value=10000
  Demux : Demux  Outputs=2
  GreaterThan : RelationalOperator  OutDataTypeStr=boolean  RndMeth=Simplest
  Nonlinear_MPC : Subsystem
  SOC ref : Constant  Value=0.5
  Terminator : Terminator
  Genset Command : Outport
  MPC Engine Power Command : Outport  Port=2
  wires:
  Power Demand/1 -> Nonlinear_MPC/3(Measured Disturbance)
  "SOC(%) "/1 -> % to num/1
  SOC ref/1 -> Nonlinear_MPC/2(SOC_ref)
  % to num/1 -> Nonlinear_MPC/1(SOC)
  Chart/1(GensetCmd) -> Genset Command/1
  Demux/2 -> GreaterThan/1, MPC Engine Power Command/1
  Constant/1 -> GreaterThan/2
  Clock/1 -> Chart/2(t)
  Nonlinear_MPC/1(Manipulated Variable) -> Demux/1
  GreaterThan/1 -> Chart/1(MPC_Decision)
  Demux/1 -> Terminator/1

== system Thesis_VehicleModel_MPC_ECMS/Driver and Vehicle Dynamics /Dynamic Model ==
  Steering input (rad) : Inport
  Drive Shaft Torque (N.m) : Inport  Port=2
  Friction Force (N) : Inport  Port=3
  Driveline : Subsystem
  Gain : Gain  Gain=3.6
  Sqrt : Sqrt  SaturateOnIntegerOverflow=on
  Square : Math  Operator=square  SaturateOnIntegerOverflow=on
  Square1 : Math  Operator=square  SaturateOnIntegerOverflow=on
  Sum : Sum  Inputs=|++
  Three Degree Bicycle Model : Subsystem
  m to mile : Gain  Gain=1/1609
  Yaw Angle Angle (rad) : Outport
  Global Velocity (km/h) : Outport  Port=2
  X coordinate (m) : Outport  Port=3
  Y coordinate (m) : Outport  Port=4
  Longitudinal Velocity (m/s) : Outport  Port=5
  Distance(mile) : Outport  Port=6
  wires:
  Gain/1 -> Global Velocity (km/h)/1  "Velocity(km/h)"
  Three Degree Bicycle Model/1(Yaw Angle) -> Yaw Angle Angle (rad)/1
  Three Degree Bicycle Model/3(X Coordinate) -> Square1/1, X coordinate (m)/1  "X"
  Three Degree Bicycle Model/5(front_slip_angle) -> Driveline/3(Front Slip)
  Three Degree Bicycle Model/6(rear_slip_angle) -> Driveline/4(Rear Slip)
  Driveline/1("Front Wheel Fx ") -> Three Degree Bicycle Model/2(Front Wheel Longitudinal Force)
  Driveline/3(Front Wheel Fy) -> Three Degree Bicycle Model/4(Front Wheel Lateral Force)
  Three Degree Bicycle Model/2(Y Coordinate) -> Square/1, Y coordinate (m)/1  "Y"
  Three Degree Bicycle Model/4(Global Velocity) -> Gain/1  "Velocity(m/s)"
  Driveline/4(Rear Wheel Fy) -> Three Degree Bicycle Model/5(Rear Wheel Lateral Force)
  Driveline/2(Rear Wheel Fx) -> Three Degree Bicycle Model/3(Rear Wheel Longitudinal Force)
  Three Degree Bicycle Model/7(Acceleration) -> Driveline/5(a)
  Driveline/5(Acceleration Explict Term Conversion) -> Three Degree Bicycle Model/6(Acceleration Explict Terms Conversion)
  Three Degree Bicycle Model/8("AeroResistance ") -> Driveline/6("AeroResistance ")
  Three Degree Bicycle Model/9("Longitudinal Velocity ") -> Driveline/7(Longitudinal Velocity), Longitudinal Velocity (m/s)/1
  Friction Force (N)/1 -> Driveline/2(Friction Brake Force)
  Steering input (rad)/1 -> Three Degree Bicycle Model/1(Steering Input)
  Drive Shaft Torque (N.m)/1 -> Driveline/1(Gearbox Output Torque)
  Square/1 -> Sum/1
  Square1/1 -> Sum/2
  Sum/1 -> Sqrt/1
  Sqrt/1 -> m to mile/1
  m to mile/1 -> Distance(mile)/1

== system Thesis_VehicleModel_MPC_ECMS/Driver and Vehicle Dynamics /EMRAX Motor Model  ==
  Longitudinal Velocity (m/s) : Inport
  "Gear " : Inport  Port=2
  APP : Inport  Port=3
  BPP : Inport  Port=4
  1-D Lookup Table1 : Lookup_n-D  NumberOfTableDimensions=1  BreakpointsForDimension1=[0,1,2,3,4,5,6]  Table=[0,4.40,2.59,1.8,1.34,1.00,0.75]  InternalRulePriority=Speed  RndMeth=Simplest  InputSameDT=on
  Brake System : Subsystem
  Bus Selector : BusSelector  OutputSignals=Friction Brake Force,Regen Brake Torque
  EMRAX 228 Motor : Subsystem
  Gain : Gain  Gain=MDL.Driveline.TFRatio/MDL.Tire.EffectiveRadius
  Product1 : Product
  Motor Torque Output (N.m) : Outport
  Power Consumption (W) : Outport  Port=2
  "Friction Force (N) " : Outport  Port=3
  wires:
  Longitudinal Velocity (m/s)/1 -> Brake System/2(V (m/s)), Gain/1
  Gain/1 -> Product1/1  "Wheel Speed"
  Product1/1 -> EMRAX 228 Motor/3(Motor Speed (rad/s))  "Motor Speed (rad/s)"
  "Gear "/1 -> 1-D Lookup Table1/1
  BPP/1 -> Brake System/1("BPP ")
  Brake System/1(BrakeCmd) -> Bus Selector/1
  Bus Selector/1 -> "Friction Force (N) "/1  "<Friction Brake Force>"
  Bus Selector/2 -> EMRAX 228 Motor/1(Regen Brake Torque Cmd)  "<Regen Brake Torque>"
  1-D Lookup Table1/1 -> Product1/2
  APP/1 -> EMRAX 228 Motor/2(APP)
  EMRAX 228 Motor/1(Motor Torque) -> Motor Torque Output (N.m)/1
  EMRAX 228 Motor/2(Power_Consumption) -> Power Consumption (W)/1

== system Thesis_VehicleModel_MPC_ECMS/Driver and Vehicle Dynamics /Transmission ==
  "Motor Shaft Torque " : Inport
  Gear : Inport  Port=2
  1-D Lookup Table1 : Lookup_n-D  NumberOfTableDimensions=1  BreakpointsForDimension1=[0,1,2,3,4,5,6]  Table=[0,4.40,2.59,1.8,1.34,1.00,0.75]  InternalRulePriority=Speed  RndMeth=Simplest  InputSameDT=on
  Product : Product
  Drive Shaft Torque : Outport
  wires:
  Gear/1 -> 1-D Lookup Table1/1
  "Motor Shaft Torque "/1 -> Product/1
  1-D Lookup Table1/1 -> Product/2
  Product/1 -> Drive Shaft Torque/1

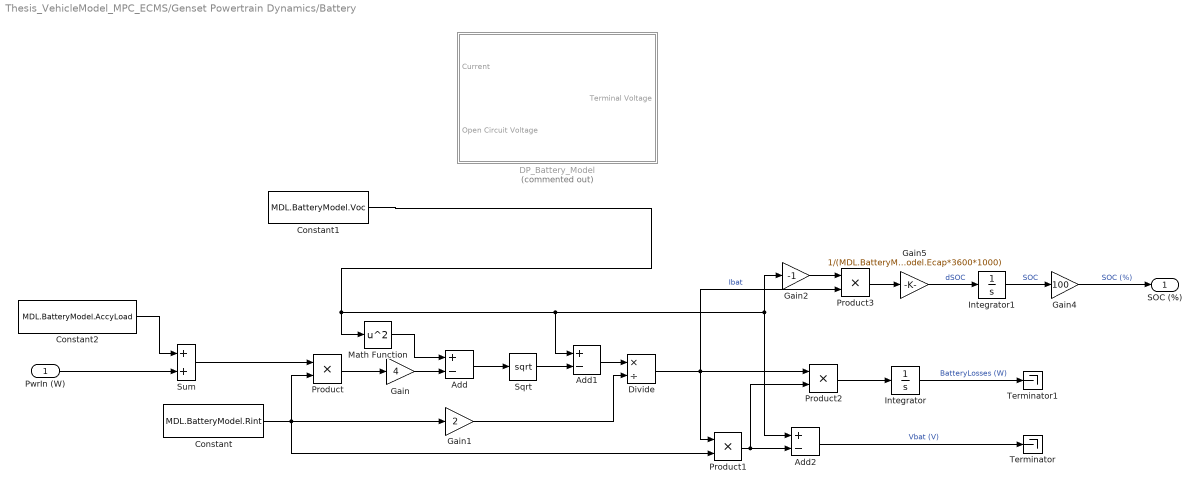
== system Thesis_VehicleModel_MPC_ECMS/Genset Powertrain Dynamics/Battery ==
  PwrIn (W) : Inport
  Add : Sum  Inputs=+-
  Add1 : Sum  Inputs=+-
  Add2 : Sum  Inputs=+-
  Constant : Constant  Value=MDL.BatteryModel.Rint
  Constant1 : Constant  Value=MDL.BatteryModel.Voc
  Constant2 : Constant  Value=MDL.BatteryModel.AccyLoad
  DP_Battery_Model : Subsystem  Commented=on
  Divide : Product  Inputs=*/
  Gain : Gain  Gain=4
  Gain1 : Gain  Gain=2
  Gain2 : Gain  Gain=-1
  Gain4 : Gain  Gain=100
  Gain5 : Gain  Gain=1/(MDL.BatteryModel.Ecap*3600*1000)
  Integrator : Integrator
  Integrator1 : Integrator  InitialCondition=MDL.BatteryModel.SOCi
  Math Function : Math  Operator=square  SaturateOnIntegerOverflow=on
  Product{,1..3} (4 alike) : Product  RndMeth=Zero
  Sqrt : Sqrt  SaturateOnIntegerOverflow=on
  Sum : Sum
  Terminator : Terminator
  Terminator1 : Terminator
  SOC (%) : Outport
  wires:
  Constant/1 -> Product/2, Gain1/1, Product1/2
  Product/1 -> Gain/1
  Constant1/1 -> Math Function/1, Add1/1, Add2/1, Gain2/1
  Math Function/1 -> Add/1
  Gain/1 -> Add/2
  Add/1 -> Sqrt/1
  Sqrt/1 -> Add1/2
  Add1/1 -> Divide/1
  Gain1/1 -> Divide/2
  Divide/1 -> Product1/1, Product2/1, Product3/2  "Ibat"
  Product1/1 -> Add2/2, Product2/2
  Product2/1 -> Integrator/1
  Gain2/1 -> Product3/1
  Product3/1 -> Gain5/1
  Constant2/1 -> Sum/1
  Sum/1 -> Product/1
  Gain4/1 -> SOC (%)/1  "SOC (%)"
  PwrIn (W)/1 -> Sum/2
  Integrator/1 -> Terminator1/1  "BatteryLosses (W)"
  Add2/1 -> Terminator/1  "Vbat (V)"
  Integrator1/1 -> Gain4/1  "SOC"
  Gain5/1 -> Integrator1/1  "dSOC"

== system Thesis_VehicleModel_MPC_ECMS/Genset Powertrain Dynamics/Engine ==
  Genset Cmd : Inport
  "Torque_Load(N) " : Inport  Port=2
  TPS Command : Inport  Port=3
  "Engine_Dynamics " : Subsystem
  Fuel_Consumption : Subsystem
  L to Gal : Gain  Gain=1/3.785
  Product : Product
  g to L : Gain  Gain=0.77/1000
  rpm2rads : Gain  Gain=pi/30
  MechPwrIn (W) : Outport
  "Eng_rpm " : Outport  Port=2
  Fuel Consumption(Gallon) : Outport  Port=3
  wires:
  Genset Cmd/1 -> Fuel_Consumption/1(Genset_Cmd)
  "Torque_Load(N) "/1 -> "Engine_Dynamics "/1("Torque_load ")
  "Engine_Dynamics "/2(Eng_rpm) -> "Eng_rpm "/1, Fuel_Consumption/4(Engine rpm), rpm2rads/1
  Fuel_Consumption/1(Fuel Consumption(g)) -> g to L/1
  Product/1 -> Fuel_Consumption/3(EngPwrOut(W)), MechPwrIn (W)/1
  rpm2rads/1 -> Product/1
  "Engine_Dynamics "/1(Engine torque) -> Product/2, Fuel_Consumption/2(Engine Torque)
  TPS Command/1 -> "Engine_Dynamics "/2(TPS Command)
  g to L/1 -> L to Gal/1
  L to Gal/1 -> Fuel Consumption(Gallon)/1

== system Thesis_VehicleModel_MPC_ECMS/Genset Powertrain Dynamics/Generator ==
  MechPwrIn(W) : Inport
  GensetCmd : Inport  Port=2
  Power Setpoint : Inport  Port=3
  Constant1 : Constant  Value=0
  Constant2 : Constant  Value=0
  Current Servo System : TransferFcn  Denominator=[0.2 1]
  Load Torque Servo System : TransferFcn  Denominator=[0.2 1]
  Product : Product
  Saturation : Saturate  UpperLimit=70  LowerLimit=0
  Saturation Dynamic : simulink/Discontinuities/Saturation Dynamic  OutMin=[]  OutMax=[]  OutDataTypeStr=Inherit: Same as second input  OutDataType=fixdt(1, 16)  OutScaling=2^-10  DoSatur=off
  Saturation Dynamic1 : simulink/Discontinuities/Saturation Dynamic  OutMin=[]  OutMax=[]  OutDataTypeStr=Inherit: Same as second input  OutDataType=fixdt(1, 16)  OutScaling=2^-10  DoSatur=off
  Saturation1 : Saturate  UpperLimit=inf  LowerLimit=0
  Subsystem : Subsystem
  Subtract : Sum  Inputs=+-
  Terminator : Terminator
  Thermal Contraint : Subsystem
  "Voltage, Current and Load Torque Mapping" : MATLAB Function  TreatAsAtomicUnit=on
  GenPwrOut (W) : Outport
  "Torque_Load " : Outport  Port=2
  MaxMechPwr : Outport  Port=3
  wires:
  GensetCmd/1 -> Subsystem/2("Genset Cmd ")
  Constant1/1 -> Saturation Dynamic/3
  Saturation Dynamic1/1 -> GenPwrOut (W)/1  "GenPwrOut (W)"
  Saturation Dynamic/1 -> Subtract/1, Subsystem/1(Mech_Pwr), Thermal Contraint/1(MechPwrIn)
  Thermal Contraint/1(MaxMechPwr) -> MaxMechPwr/1, Saturation Dynamic/1
  MechPwrIn(W)/1 -> Saturation Dynamic/2
  Subsystem/1(Pwr_Loss) -> Subtract/2  "Gen Pwr Loss"
  "Voltage, Current and Load Torque Mapping"/3(LoadTorque) -> Saturation/1  "T_load*"
  Load Torque Servo System/1 -> "Torque_Load "/1  "T_load"
  "Voltage, Current and Load Torque Mapping"/2(Current) -> Current Servo System/1  "Current*"
  Power Setpoint/1 -> "Voltage, Current and Load Torque Mapping"/1(P)  "Power_cmd"
  Saturation/1 -> Load Torque Servo System/1
  Constant2/1 -> Saturation Dynamic1/3
  Product/1 -> Saturation Dynamic1/2
  "Voltage, Current and Load Torque Mapping"/1(Volt) -> Product/2
  Current Servo System/1 -> Terminator/1, Product/1  "Current"
  Subtract/1 -> Saturation1/1
  Saturation1/1 -> Saturation Dynamic1/1  "Gen Upper Bound"

== system Thesis_VehicleModel_MPC_ECMS/Genset Powertrain Dynamics/Power//rpm Setpoints ==
  Power Command : Inport
  Genset Cmd : Inport  Port=2
  Chart : Stateflow chart  TreatAsAtomicUnit=on
  Clock : Clock
  MATLAB Function : MATLAB Function  TreatAsAtomicUnit=on
  Power Setpoint : Outport
  rpm Setpoint : Outport  Port=2
  wires:
  Power Command/1 -> MATLAB Function/1(Power_Cmd)
  Clock/1 -> Chart/2(t)
  MATLAB Function/1(PowerSetPoint) -> Chart/1(PowerSetPoint)
  MATLAB Function/2(rpmSetPoint) -> Chart/3(rpmSetPoint)
  Chart/2(PowerCmd) -> Power Setpoint/1
  Chart/1(rpmCmd) -> rpm Setpoint/1
  Genset Cmd/1 -> MATLAB Function/2(GensetCmd)

== system Thesis_VehicleModel_MPC_ECMS/Genset Powertrain Dynamics/Rpm Controller ==
  Engine rpm : Inport
  rpm setpoint : Inport  Port=2
  Engine Power Set Point : Inport  Port=3
  Calculate Feedback Mapping : Product  Multiplication=Matrix(*)
  Calculate Fix Point : Subsystem
  Demux : Demux  Outputs=2
  Gain : Gain  Gain=30/pi
  Kalman Filter : Subsystem
  LQG Gain Mapping : MATLAB Function  TreatAsAtomicUnit=on
  Noise : RandomNumber  Variance=300  SampleTime=0.1
  Scope : Scope
  Scope1 : Scope
  Sum : Sum  Inputs=|-+
  Sum1 : Sum  Inputs=|++
  Sum2 : Sum  Inputs=|++
  TPS limit : Saturate  UpperLimit=0.98  LowerLimit=0
  Terminator : Terminator
  dSPACE CANBUS Protocol : Subsystem  Commented=on
  rpm regulation : Stateflow chart  Commented=on  TreatAsAtomicUnit=on
  rpm2rads1 : Gain  Gain=pi/30
  TPS Command : Outport
  wires:
  Sum2/1 -> LQG Gain Mapping/1(rpm), rpm2rads1/1, Kalman Filter/2("rpm ")  "Engine rpm with noise"
  Kalman Filter/1("x_hat ") -> Scope/1, Sum/2, Gain/1  "State Estimation x_hat"
  Sum/1 -> Calculate Feedback Mapping/2
  Sum1/1 -> Kalman Filter/3(u)
  rpm2rads1/1 -> Kalman Filter/1(y)
  TPS limit/1 -> Sum1/2, TPS Command/1
  LQG Gain Mapping/2(gain) -> Calculate Feedback Mapping/1
  Engine rpm/1 -> Sum2/1
  Noise/1 -> Sum2/2
  LQG Gain Mapping/1(comp) -> Sum1/1
  rpm setpoint/1 -> Calculate Fix Point/1(rpm set point)
  Calculate Fix Point/1(rpm_cmd) -> LQG Gain Mapping/2(rpm_cmd)
  Calculate Fix Point/2(fix point (2 states)) -> Sum/1
  Engine Power Set Point/1 -> LQG Gain Mapping/3(PowerSetPoint)
  Calculate Feedback Mapping/1 -> TPS limit/1
  Gain/1 -> Demux/1
  Demux/1 -> Scope1/1
  Demux/2 -> Terminator/1

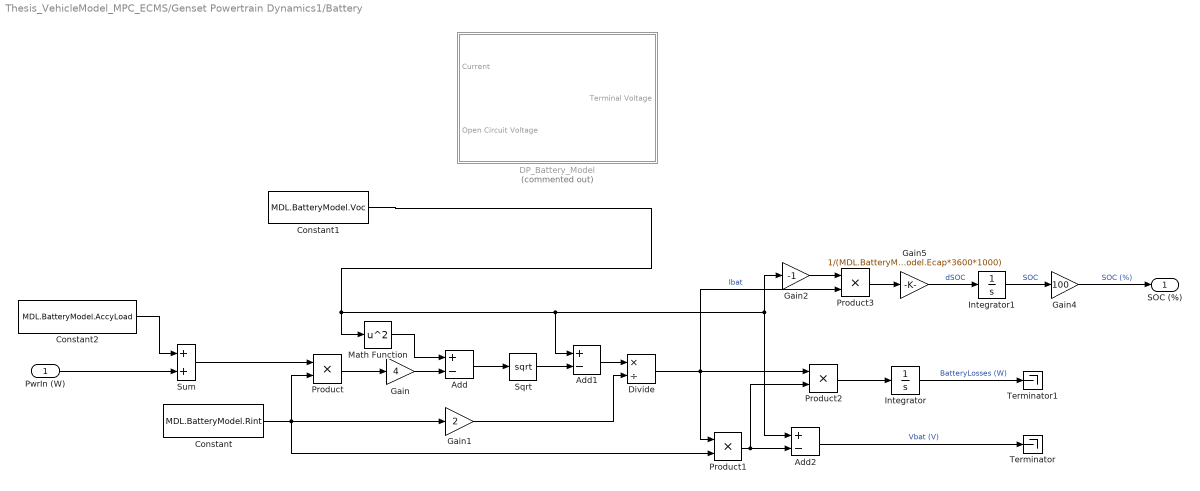
== system Thesis_VehicleModel_MPC_ECMS/Genset Powertrain Dynamics1/Battery ==
  PwrIn (W) : Inport
  Add : Sum  Inputs=+-
  Add1 : Sum  Inputs=+-
  Add2 : Sum  Inputs=+-
  Constant : Constant  Value=MDL.BatteryModel.Rint
  Constant1 : Constant  Value=MDL.BatteryModel.Voc
  Constant2 : Constant  Value=MDL.BatteryModel.AccyLoad
  DP_Battery_Model : Subsystem  Commented=on
  Divide : Product  Inputs=*/
  Gain : Gain  Gain=4
  Gain1 : Gain  Gain=2
  Gain2 : Gain  Gain=-1
  Gain4 : Gain  Gain=100
  Gain5 : Gain  Gain=1/(MDL.BatteryModel.Ecap*3600*1000)
  Integrator : Integrator
  Integrator1 : Integrator  InitialCondition=MDL.BatteryModel.SOCi
  Math Function : Math  Operator=square  SaturateOnIntegerOverflow=on
  Product{,1..3} (4 alike) : Product  RndMeth=Zero
  Sqrt : Sqrt  SaturateOnIntegerOverflow=on
  Sum : Sum
  Terminator : Terminator
  Terminator1 : Terminator
  SOC (%) : Outport
  wires:
  Constant/1 -> Product/2, Gain1/1, Product1/2
  Product/1 -> Gain/1
  Constant1/1 -> Math Function/1, Add1/1, Add2/1, Gain2/1
  Math Function/1 -> Add/1
  Gain/1 -> Add/2
  Add/1 -> Sqrt/1
  Sqrt/1 -> Add1/2
  Add1/1 -> Divide/1
  Gain1/1 -> Divide/2
  Divide/1 -> Product1/1, Product2/1, Product3/2  "Ibat"
  Product1/1 -> Add2/2, Product2/2
  Product2/1 -> Integrator/1
  Gain2/1 -> Product3/1
  Product3/1 -> Gain5/1
  Constant2/1 -> Sum/1
  Sum/1 -> Product/1
  Gain4/1 -> SOC (%)/1  "SOC (%)"
  PwrIn (W)/1 -> Sum/2
  Integrator/1 -> Terminator1/1  "BatteryLosses (W)"
  Add2/1 -> Terminator/1  "Vbat (V)"
  Integrator1/1 -> Gain4/1  "SOC"
  Gain5/1 -> Integrator1/1  "dSOC"

== system Thesis_VehicleModel_MPC_ECMS/Genset Powertrain Dynamics1/Engine ==
  Genset Cmd : Inport
  "Torque_Load(N) " : Inport  Port=2
  TPS Command : Inport  Port=3
  "Engine_Dynamics " : Subsystem
  Fuel_Consumption : Subsystem
  L to Gal : Gain  Gain=1/3.785
  Product : Product
  g to L : Gain  Gain=0.77/1000
  rpm2rads : Gain  Gain=pi/30
  MechPwrIn (W) : Outport
  "Eng_rpm " : Outport  Port=2
  Fuel Consumption(Gallon) : Outport  Port=3
  wires:
  Genset Cmd/1 -> Fuel_Consumption/1(Genset_Cmd)
  "Torque_Load(N) "/1 -> "Engine_Dynamics "/1("Torque_load ")
  "Engine_Dynamics "/2(Eng_rpm) -> "Eng_rpm "/1, Fuel_Consumption/4(Engine rpm), rpm2rads/1
  Fuel_Consumption/1(Fuel Consumption(g)) -> g to L/1
  Product/1 -> Fuel_Consumption/3(EngPwrOut(W)), MechPwrIn (W)/1
  rpm2rads/1 -> Product/1
  "Engine_Dynamics "/1(Engine torque) -> Product/2, Fuel_Consumption/2(Engine Torque)
  TPS Command/1 -> "Engine_Dynamics "/2(TPS Command)
  g to L/1 -> L to Gal/1
  L to Gal/1 -> Fuel Consumption(Gallon)/1

== system Thesis_VehicleModel_MPC_ECMS/Genset Powertrain Dynamics1/Generator ==
  MechPwrIn(W) : Inport
  GensetCmd : Inport  Port=2
  Power Setpoint : Inport  Port=3
  Constant1 : Constant  Value=0
  Constant2 : Constant  Value=0
  Current Servo System : TransferFcn  Denominator=[0.2 1]
  Load Torque Servo System : TransferFcn  Denominator=[0.2 1]
  Product : Product
  Saturation : Saturate  UpperLimit=70  LowerLimit=0
  Saturation Dynamic : simulink/Discontinuities/Saturation Dynamic  OutMin=[]  OutMax=[]  OutDataTypeStr=Inherit: Same as second input  OutDataType=fixdt(1, 16)  OutScaling=2^-10  DoSatur=off
  Saturation Dynamic1 : simulink/Discontinuities/Saturation Dynamic  OutMin=[]  OutMax=[]  OutDataTypeStr=Inherit: Same as second input  OutDataType=fixdt(1, 16)  OutScaling=2^-10  DoSatur=off
  Saturation1 : Saturate  UpperLimit=inf  LowerLimit=0
  Subsystem : Subsystem
  Subtract : Sum  Inputs=+-
  Terminator : Terminator
  Thermal Contraint : Subsystem
  "Voltage, Current and Load Torque Mapping" : MATLAB Function  TreatAsAtomicUnit=on
  GenPwrOut (W) : Outport
  "Torque_Load " : Outport  Port=2
  MaxMechPwr : Outport  Port=3
  wires:
  GensetCmd/1 -> Subsystem/2("Genset Cmd ")
  Constant1/1 -> Saturation Dynamic/3
  Saturation Dynamic1/1 -> GenPwrOut (W)/1  "GenPwrOut (W)"
  Saturation Dynamic/1 -> Subtract/1, Subsystem/1(Mech_Pwr), Thermal Contraint/1(MechPwrIn)
  Thermal Contraint/1(MaxMechPwr) -> MaxMechPwr/1, Saturation Dynamic/1
  MechPwrIn(W)/1 -> Saturation Dynamic/2
  Subsystem/1(Pwr_Loss) -> Subtract/2  "Gen Pwr Loss"
  "Voltage, Current and Load Torque Mapping"/3(LoadTorque) -> Saturation/1  "T_load*"
  Load Torque Servo System/1 -> "Torque_Load "/1  "T_load"
  "Voltage, Current and Load Torque Mapping"/2(Current) -> Current Servo System/1  "Current*"
  Power Setpoint/1 -> "Voltage, Current and Load Torque Mapping"/1(P)  "Power_cmd"
  Saturation/1 -> Load Torque Servo System/1
  Constant2/1 -> Saturation Dynamic1/3
  Product/1 -> Saturation Dynamic1/2
  "Voltage, Current and Load Torque Mapping"/1(Volt) -> Product/2
  Current Servo System/1 -> Terminator/1, Product/1  "Current"
  Subtract/1 -> Saturation1/1
  Saturation1/1 -> Saturation Dynamic1/1  "Gen Upper Bound"

== system Thesis_VehicleModel_MPC_ECMS/Genset Powertrain Dynamics1/Power//rpm Setpoints ==
  Power Command : Inport
  Genset Cmd : Inport  Port=2
  Chart : Stateflow chart  TreatAsAtomicUnit=on
  Clock : Clock
  MATLAB Function : MATLAB Function  TreatAsAtomicUnit=on
  Power Setpoint : Outport
  rpm Setpoint : Outport  Port=2
  wires:
  Power Command/1 -> MATLAB Function/1(Power_Cmd)
  Clock/1 -> Chart/2(t)
  MATLAB Function/1(PowerSetPoint) -> Chart/1(PowerSetPoint)
  MATLAB Function/2(rpmSetPoint) -> Chart/3(rpmSetPoint)
  Chart/2(PowerCmd) -> Power Setpoint/1
  Chart/1(rpmCmd) -> rpm Setpoint/1
  Genset Cmd/1 -> MATLAB Function/2(GensetCmd)

== system Thesis_VehicleModel_MPC_ECMS/Genset Powertrain Dynamics1/Rpm Controller ==
  Engine rpm : Inport
  rpm setpoint : Inport  Port=2
  Engine Power Set Point : Inport  Port=3
  Calculate Feedback Mapping : Product  Multiplication=Matrix(*)
  Calculate Fix Point : Subsystem
  Demux : Demux  Outputs=2
  Gain : Gain  Gain=30/pi
  Kalman Filter : Subsystem
  LQG Gain Mapping : MATLAB Function  TreatAsAtomicUnit=on
  Noise : RandomNumber  Variance=300  SampleTime=0.1
  Scope : Scope
  Scope1 : Scope
  Sum : Sum  Inputs=|-+
  Sum1 : Sum  Inputs=|++
  Sum2 : Sum  Inputs=|++
  TPS limit : Saturate  UpperLimit=0.98  LowerLimit=0
  Terminator : Terminator
  dSPACE CANBUS Protocol : Subsystem  Commented=on
  rpm regulation : Stateflow chart  Commented=on  TreatAsAtomicUnit=on
  rpm2rads1 : Gain  Gain=pi/30
  TPS Command : Outport
  wires:
  Sum2/1 -> LQG Gain Mapping/1(rpm), rpm2rads1/1, Kalman Filter/2("rpm ")  "Engine rpm with noise"
  Kalman Filter/1("x_hat ") -> Scope/1, Sum/2, Gain/1  "State Estimation x_hat"
  Sum/1 -> Calculate Feedback Mapping/2
  Sum1/1 -> Kalman Filter/3(u)
  rpm2rads1/1 -> Kalman Filter/1(y)
  TPS limit/1 -> Sum1/2, TPS Command/1
  LQG Gain Mapping/2(gain) -> Calculate Feedback Mapping/1
  Engine rpm/1 -> Sum2/1
  Noise/1 -> Sum2/2
  LQG Gain Mapping/1(comp) -> Sum1/1
  rpm setpoint/1 -> Calculate Fix Point/1(rpm set point)
  Calculate Fix Point/1(rpm_cmd) -> LQG Gain Mapping/2(rpm_cmd)
  Calculate Fix Point/2(fix point (2 states)) -> Sum/1
  Engine Power Set Point/1 -> LQG Gain Mapping/3(PowerSetPoint)
  Calculate Feedback Mapping/1 -> TPS limit/1
  Gain/1 -> Demux/1
  Demux/1 -> Scope1/1
  Demux/2 -> Terminator/1

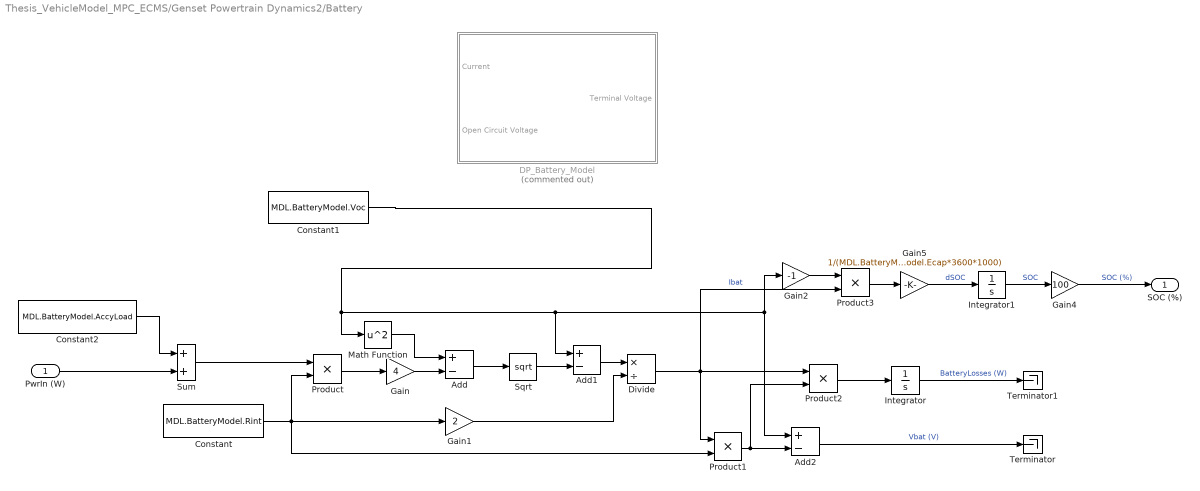
== system Thesis_VehicleModel_MPC_ECMS/Genset Powertrain Dynamics2/Battery ==
  PwrIn (W) : Inport
  Add : Sum  Inputs=+-
  Add1 : Sum  Inputs=+-
  Add2 : Sum  Inputs=+-
  Constant : Constant  Value=MDL.BatteryModel.Rint
  Constant1 : Constant  Value=MDL.BatteryModel.Voc
  Constant2 : Constant  Value=MDL.BatteryModel.AccyLoad
  DP_Battery_Model : Subsystem  Commented=on
  Divide : Product  Inputs=*/
  Gain : Gain  Gain=4
  Gain1 : Gain  Gain=2
  Gain2 : Gain  Gain=-1
  Gain4 : Gain  Gain=100
  Gain5 : Gain  Gain=1/(MDL.BatteryModel.Ecap*3600*1000)
  Integrator : Integrator
  Integrator1 : Integrator  InitialCondition=MDL.BatteryModel.SOCi
  Math Function : Math  Operator=square  SaturateOnIntegerOverflow=on
  Product{,1..3} (4 alike) : Product  RndMeth=Zero
  Sqrt : Sqrt  SaturateOnIntegerOverflow=on
  Sum : Sum
  Terminator : Terminator
  Terminator1 : Terminator
  SOC (%) : Outport
  wires:
  Constant/1 -> Product/2, Gain1/1, Product1/2
  Product/1 -> Gain/1
  Constant1/1 -> Math Function/1, Add1/1, Add2/1, Gain2/1
  Math Function/1 -> Add/1
  Gain/1 -> Add/2
  Add/1 -> Sqrt/1
  Sqrt/1 -> Add1/2
  Add1/1 -> Divide/1
  Gain1/1 -> Divide/2
  Divide/1 -> Product1/1, Product2/1, Product3/2  "Ibat"
  Product1/1 -> Add2/2, Product2/2
  Product2/1 -> Integrator/1
  Gain2/1 -> Product3/1
  Product3/1 -> Gain5/1
  Constant2/1 -> Sum/1
  Sum/1 -> Product/1
  Gain4/1 -> SOC (%)/1  "SOC (%)"
  PwrIn (W)/1 -> Sum/2
  Integrator/1 -> Terminator1/1  "BatteryLosses (W)"
  Add2/1 -> Terminator/1  "Vbat (V)"
  Integrator1/1 -> Gain4/1  "SOC"
  Gain5/1 -> Integrator1/1  "dSOC"

== system Thesis_VehicleModel_MPC_ECMS/Genset Powertrain Dynamics2/Engine ==
  Genset Cmd : Inport
  "Torque_Load(N) " : Inport  Port=2
  TPS Command : Inport  Port=3
  "Engine_Dynamics " : Subsystem
  Fuel_Consumption : Subsystem
  L to Gal : Gain  Gain=1/3.785
  Product : Product
  g to L : Gain  Gain=0.77/1000
  rpm2rads : Gain  Gain=pi/30
  MechPwrIn (W) : Outport
  "Eng_rpm " : Outport  Port=2
  Fuel Consumption(Gallon) : Outport  Port=3
  wires:
  Genset Cmd/1 -> Fuel_Consumption/1(Genset_Cmd)
  "Torque_Load(N) "/1 -> "Engine_Dynamics "/1("Torque_load ")
  "Engine_Dynamics "/2(Eng_rpm) -> "Eng_rpm "/1, Fuel_Consumption/4(Engine rpm), rpm2rads/1
  Fuel_Consumption/1(Fuel Consumption(g)) -> g to L/1
  Product/1 -> Fuel_Consumption/3(EngPwrOut(W)), MechPwrIn (W)/1
  rpm2rads/1 -> Product/1
  "Engine_Dynamics "/1(Engine torque) -> Product/2, Fuel_Consumption/2(Engine Torque)
  TPS Command/1 -> "Engine_Dynamics "/2(TPS Command)
  g to L/1 -> L to Gal/1
  L to Gal/1 -> Fuel Consumption(Gallon)/1
